simulink model "sh"  (Simulink 8.6)
settings: Solver=FixedStepDiscrete  StartTime=0.0  StopTime=t_sim  FixedStep=ts  RelTol=1e-3
values from neighbouring files (symbols this model uses):
  ts = 0.000001    (= 1e-06)    [main.m]
settings Model: Creator=mailly  LastModifiedBy=mailly
settings OptimizationCC: ExpressionDepthLimit=128  InitFltsAndDblsToZero=on
settings DebuggingCC: SaveWithParameterizedLinksMsg=none  SignalResolutionControl=TryResolveAllWithWarning  MultiTaskDSMMsg=warning  MultiTaskCondExecSysMsg=none  FcnCallInpInsideContextMsg=UseLocalSettings  StateNameClashWarn=none
settings GRTTargetCC: TargetFcnLib=ansi_tfl_tmw.mat  GeneratePreprocessorConditionals=Use local settings

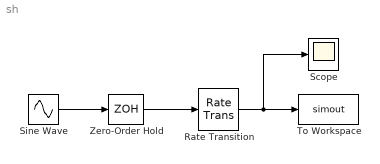
== system sh ==
  Rate Transition : RateTransition
  Scope : Scope
  Sine Wave : Sin  Frequency=2*pi*100  SampleTime=0
  To Workspace : ToWorkspace  VariableName=simout  SampleTime=ts
  Zero-Order Hold : ZeroOrderHold  SampleTime=0.001
  wires:
  Sine Wave/1 -> Zero-Order Hold/1
  Zero-Order Hold/1 -> Rate Transition/1
  Rate Transition/1 -> To Workspace/1, Scope/1
